simulink model "sim1"  (R2024a)
settings: Solver=FixedStepAuto  StartTime=0.0  StopTime=3.0  FixedStep=1e-3  RelTol=1e-3
settings Model: Creator=alexe  LastModifiedBy=alexe

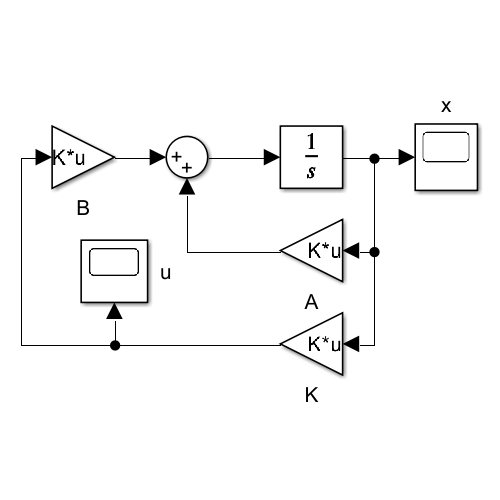
[thumbnail: Simulink's stored preview of the top-level diagram]
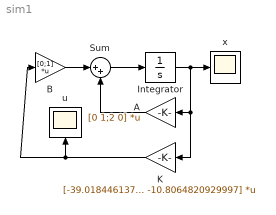
== system sim1 ==
  A : Gain  Gain=[0 1;2 0]  Multiplication=Matrix(K*u)
  B : Gain  Gain=[0;1]  Multiplication=Matrix(K*u)
  Integrator : Integrator  InitialCondition=[1; 1];
  K : Gain  Gain=[-39.0184461373194 -10.8064820929997]  Multiplication=Matrix(K*u)
  Sum : Sum  Inputs=|++
  u : Scope
  x : Scope
  wires:
  Integrator/1 -> x/1, K/1, A/1
  A/1 -> Sum/2
  B/1 -> Sum/1
  Sum/1 -> Integrator/1
  K/1 -> u/1, B/1
